simulink model "SVPWM"  (R2023b)
settings: Solver=FixedStepAuto  StartTime=0.0  StopTime=10.0  FixedStep=1e-4  RelTol=1e-3
values from neighbouring files (symbols this model uses):
  flux = 0.016884    [SVPWM.sldd]
  Period = 8000.0    [SVPWM.sldd]
  Pn = 4.0    [SVPWM.sldd]
  Udc = 24.0    [SVPWM.sldd]
libraries: mcbplantlib x1, autolibpmsmexterior x1
settings Model: DataDictionary=SVPWM.sldd  Creator=Administrator  LastModifiedBy=SkyLin
settings OptimizationCC: DefaultParameterBehavior=Inlined  UseDivisionForNetSlopeComputation=on  GainParamInheritBuiltInType=on  UseFloatMulNetSlope=on  InlineInvariantSignals=on  PassReuseOutputArgsAs=Individual arguments  ZeroExternalMemoryAtStartup=off  ZeroInternalMemoryAtStartup=off  NoFixptDivByZeroProtection=on  EfficientFloat2IntCast=on  LifeSpan=1  OptimizeBlockOrder=speed  DifferentSizesBufferReuse=on  EfficientTunableParamExpr=on
settings DebuggingCC: ParameterTunabilityLossMsg=error  UnconnectedInputMsg=warning  UnconnectedOutputMsg=warning  UnconnectedLineMsg=warning
settings HardwareCC: ProdBitPerPointer=32  ProdBitPerSizeT=32  ProdBitPerPtrDiffT=32  ProdLargestAtomicInteger=Long  ProdLargestAtomicFloat=Double  ProdWordSize=32  ProdLongLongMode=on  ProdHWDeviceType=ARM Compatible->ARM Cortex-M
settings ModelReferenceCC: EnableRefExpFcnMdlSchedulingChecks=on
settings SFSimCC: MATLABDynamicMemAlloc=off
settings RTWCC: Description=Embedded Coder  SystemTargetFile=ert.tlc  GenCodeOnly=on  TemplateMakefile=ert_default_tmf  GenerateReport=on  LaunchReport=on  GenerateCodeReplacementReport=on  DLArmComputeVersion=19.05
settings CodeAppCC: ForceParamTrailComments=on  IgnoreCustomStorageClasses=off  OperatorAnnotations=on  SimulinkDataObjDesc=on  SFDataObjDesc=on  CustomSymbolStrGlobalVar=rt$N$M  CustomSymbolStrType=$N$M  CustomSymbolStrFcn=$N$M$F  CustomSymbolStrMacro=$N$M  InsertBlockDesc=on
settings ERTTargetCC: TargetLangStandard=C99 (ISO)  CodeReplacementLibrary=ARM Cortex-M  GenerateSampleERTMain=on  IncludeMdlTerminateFcn=off  CombineSignalStateStructs=on  SuppressErrorStatus=on  SupportAbsoluteTime=off  SupportNonFinite=off  SupportComplex=off  InlinedParameterPlacement=NonHierarchical  ERTCustomFileTemplate=example_file_process.tlc  ERTFilePackagingFormat=CompactWithDataFile

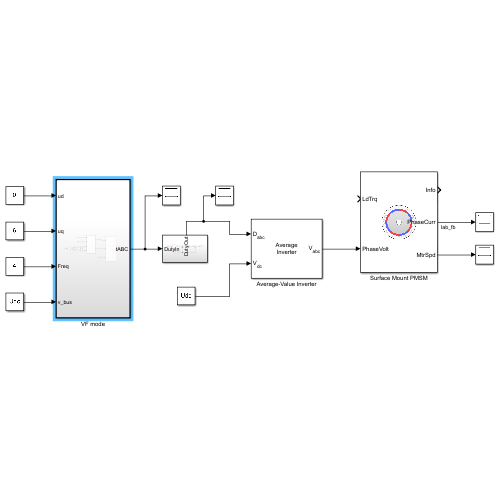
[thumbnail: Simulink's stored preview of the top-level diagram]
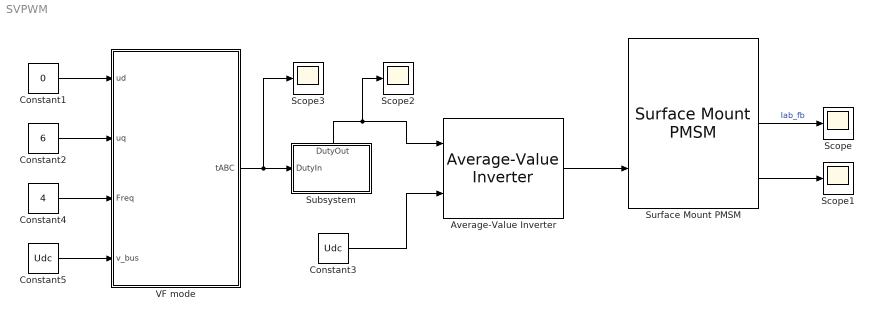
== system SVPWM ==
  Average-Value Inverter : mcbplantlib/Average-Value Inverter
  Constant1 : Constant  Value=0  OutDataTypeStr=single
  Constant2 : Constant  Value=6  OutDataTypeStr=single
  Constant3 : Constant  Value=Udc
  Constant4 : Constant  Value=4  OutDataTypeStr=single
  Constant5 : Constant  Value=Udc  OutDataTypeStr=single
  Scope{,1..3} (4 alike) : Scope
  Subsystem : Subsystem
      settings: PortSchema="{\"entries\":[{\"content\":{\"sides\":[{\"content\":{\"connectorIds\":[\"In1\"]},\"type\":\"ConnectorPlacement.EquallySpacedRectSide\",\"uuid\":\"8ccc51de-fa2a-4900-80a3-4cdf9aa76f01\"},{\"content\":{\"connectorIds\":[],\"side\":\"RIGHT\"},\"type\":\"ConnectorPlacement.EquallySpacedRectSide\",\"uuid\":\"32c06e0d-3f1d-4948-af96-e310e54308a0\"},{\"content\":{\"connectorIds\":[\"Out1\"],\"side\":\"TOP\"},\"type\":\"ConnectorPlacement.EquallySpacedRectSide\",\"uuid\":\"a9066067-2c54-42a8-b4d7-fb86ac71b860\"}]},\"type\":\"ConnectorPlacement.EquallySpacedConnector\",\"uuid\":\"e4576975-acad-4e16-822f-2c2e7f23d7a7\"}],\"packageUris\":[\"http://schema.mathworks.com/mf0/Connector/R2020b\"],\"version\":\"1.0\"}"
  Surface Mount PMSM : autolibpmsmexterior/Surface Mount PMSM  port_config=Torque  sim_type=Discrete  Ts=1e-4  P=Pn  Rs=Rs  Ldq_=L  KConstText=Permanent flux linkage constant (lambda_pm):  lambda_pm=flux  Ke=0.0059268  Kt=0.061  mechanical=[75e-6, 8e-5, 0]  idq0=[0 0]  theta_init=4/5  omega_init=0  KConst=flux  lambda_pm_calc=flux  RefBlkName='autolibpmsmexterior/Surface Mount PMSM'  aMode=5  Ldq="[0.0017      0.0017]"
  VF mode : Subsystem  TreatAsAtomicUnit=on
      settings: RTWSystemCode=Nonreusable function
  wires:
  VF mode/1(tABC) -> Scope3/1, Subsystem/1(DutyIn)
  Constant3/1 -> Average-Value Inverter/2
  Subsystem/1(DutyOut) -> Scope2/1, Average-Value Inverter/1
  Average-Value Inverter/1 -> Surface Mount PMSM/2
  Surface Mount PMSM/2 -> Scope/1  "Iab_fb"
  Surface Mount PMSM/3 -> Scope1/1
  Constant1/1 -> VF mode/1(ud)
  Constant2/1 -> VF mode/2(uq)
  Constant4/1 -> VF mode/3(Freq)
  Constant5/1 -> VF mode/4(v_bus)

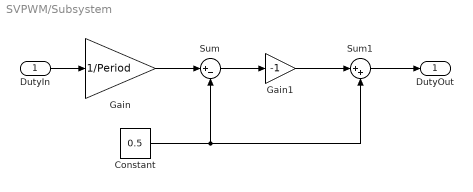
== system SVPWM/Subsystem ==
  DutyIn : Inport
  Constant : Constant  Value=0.5  SampleTime=-1
  Gain : Gain  Gain=1/Period  ParamDataTypeStr=single
  Gain1 : Gain  Gain=-1
  Sum : Sum  Inputs=|+-
  Sum1 : Sum  Inputs=|++
  DutyOut : Outport
  wires:
  Sum/1 -> Gain1/1
  Constant/1 -> Sum1/2, Sum/2
  DutyIn/1 -> Gain/1
  Gain1/1 -> Sum1/1
  Sum1/1 -> DutyOut/1
  Gain/1 -> Sum/1

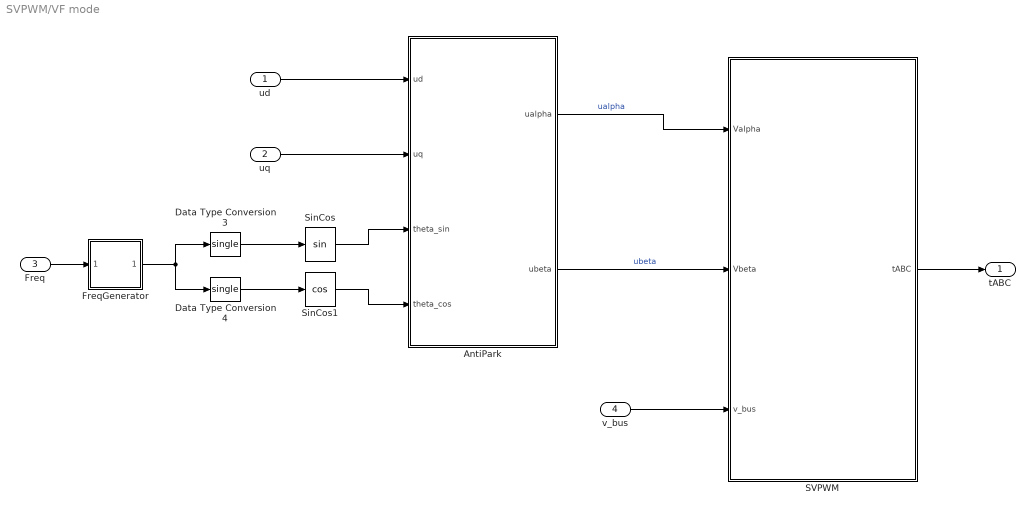
== system SVPWM/VF mode ==
  ud : Inport
  uq : Inport  Port=2
  Freq : Inport  Port=3
  v_bus : Inport  Port=4
  AntiPark : Subsystem
  Data Type Conversion3 : DataTypeConversion  OutDataTypeStr=single  SaturateOnIntegerOverflow=off  RndMeth=Floor
  Data Type Conversion4 : DataTypeConversion  OutDataTypeStr=single  SaturateOnIntegerOverflow=off  RndMeth=Floor
  FreqGenerator : Subsystem
  SVPWM : Subsystem  TreatAsAtomicUnit=on
  SinCos : Trigonometry
  SinCos1 : Trigonometry  Operator=cos
  tABC : Outport
  wires:
  FreqGenerator/1(Theta) -> Data Type Conversion4/1, Data Type Conversion3/1
  SinCos1/1 -> AntiPark/4(theta_cos)
  Data Type Conversion4/1 -> SinCos1/1
  SinCos/1 -> AntiPark/3(theta_sin)
  Freq/1 -> FreqGenerator/1(Freq)
  Data Type Conversion3/1 -> SinCos/1
  AntiPark/1(ualpha) -> SVPWM/1(Valpha)  "ualpha"
  AntiPark/2(ubeta) -> SVPWM/2(Vbeta)  "ubeta"
  ud/1 -> AntiPark/1(ud)
  uq/1 -> AntiPark/2(uq)
  v_bus/1 -> SVPWM/3(v_bus)
  SVPWM/1(tABC) -> tABC/1

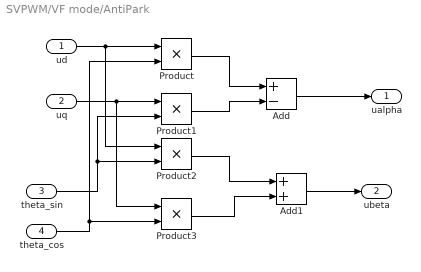
== system SVPWM/VF mode/AntiPark ==
  ud : Inport
  uq : Inport  Port=2
  theta_sin : Inport  Port=3
  theta_cos : Inport  Port=4
  Add : Sum  Inputs=+-
  Add1 : Sum
  Product{,1..3} (4 alike) : Product
  ualpha : Outport  OutDataTypeStr=single
  ubeta : Outport  Port=2  OutDataTypeStr=single
  wires:
  Add1/1 -> ubeta/1
  Product1/1 -> Add/2
  uq/1 -> Product3/1, Product1/1
  theta_cos/1 -> Product/2, Product3/2
  theta_sin/1 -> Product2/2, Product1/2
  ud/1 -> Product2/1, Product/1
  Product3/1 -> Add1/2
  Add/1 -> ualpha/1
  Product/1 -> Add/1
  Product2/1 -> Add1/1

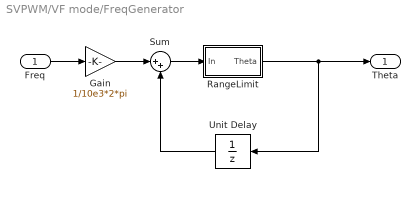
== system SVPWM/VF mode/FreqGenerator ==
  Freq : Inport
  Gain : Gain  Gain=1/10e3*2*pi  OutDataTypeStr=single
  RangeLimit : Subsystem
  Sum : Sum  Inputs=|++  OutDataTypeStr=Inherit: Same as first input
  Unit Delay : UnitDelay  SampleTime=-1  HasFrameUpgradeWarning=on
  Theta : Outport
  wires:
  Freq/1 -> Gain/1
  RangeLimit/1(Theta) -> Theta/1, Unit Delay/1
  Gain/1 -> Sum/1
  Sum/1 -> RangeLimit/1(In)
  Unit Delay/1 -> Sum/2

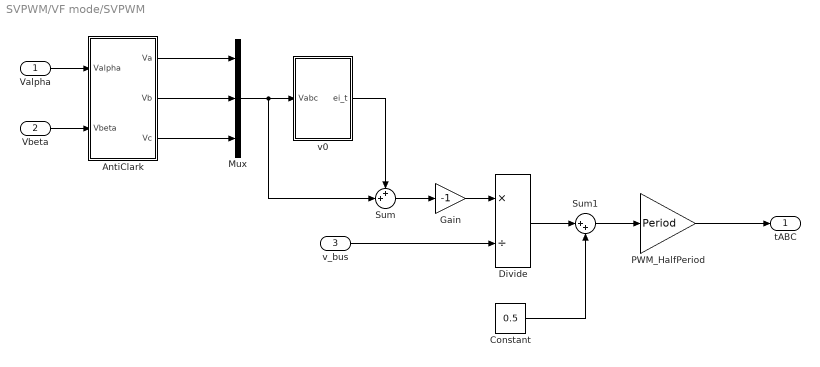
== system SVPWM/VF mode/SVPWM ==
  Valpha : Inport  OutDataTypeStr=single
  Vbeta : Inport  Port=2  OutDataTypeStr=single
  v_bus : Inport  Port=3  OutDataTypeStr=single
  AntiClark : Subsystem
  Constant : Constant  Value=0.5  OutDataTypeStr=single
  Divide : Product  Inputs=*/  OutDataTypeStr=single
  Gain : Gain  Gain=-1  OutDataTypeStr=single
  Mux : Mux  Inputs=3
  PWM_HalfPeriod : Gain  Gain=Period  OutDataTypeStr=single
  Sum : Sum  Inputs=++|  OutDataTypeStr=single
  Sum1 : Sum  Inputs=|++  OutDataTypeStr=single
  v0 : Subsystem
  tABC : Outport  OutDataTypeStr=single
  wires:
  Valpha/1 -> AntiClark/1(Valpha)
  Vbeta/1 -> AntiClark/2(Vbeta)
  v0/1(ei_t) -> Sum/1
  AntiClark/1(Va) -> Mux/1
  AntiClark/2(Vb) -> Mux/2
  AntiClark/3(Vc) -> Mux/3
  Sum/1 -> Gain/1
  Mux/1 -> Sum/2, v0/1(Vabc)
  Divide/1 -> Sum1/1
  Constant/1 -> Sum1/2
  Sum1/1 -> PWM_HalfPeriod/1
  PWM_HalfPeriod/1 -> tABC/1
  v_bus/1 -> Divide/2
  Gain/1 -> Divide/1

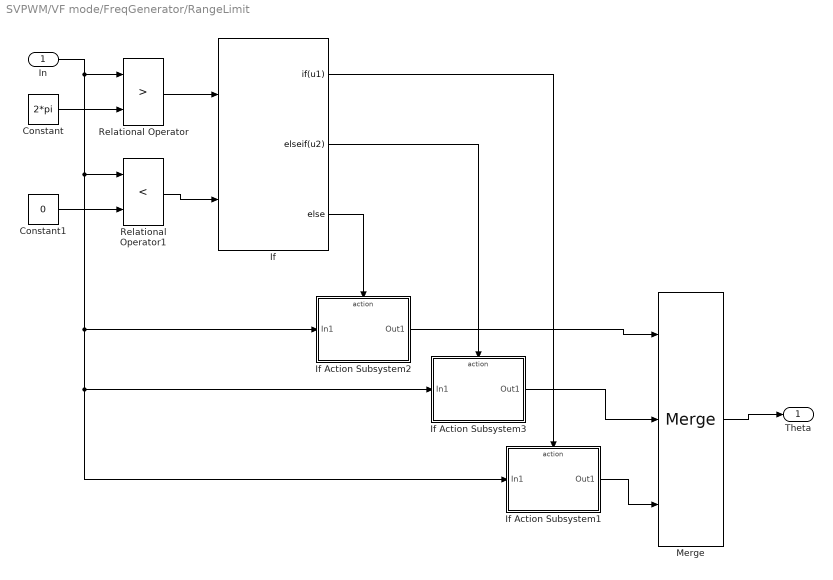
== system SVPWM/VF mode/FreqGenerator/RangeLimit ==
  In : Inport
  Constant : Constant  Value=2*pi  OutDataTypeStr=single  SampleTime=-1
  Constant1 : Constant  Value=0  OutDataTypeStr=single  SampleTime=-1
  If : If  NumInputs=2  IfExpression=u1  ElseIfExpressions=u2
  If Action Subsystem1 : Subsystem  TreatAsAtomicUnit=on
  If Action Subsystem2 : Subsystem  TreatAsAtomicUnit=on
  If Action Subsystem3 : Subsystem  TreatAsAtomicUnit=on
  Merge : Merge  Inputs=3
  Relational Operator : RelationalOperator  Operator=>  OutDataTypeStr=boolean  RndMeth=Simplest  InputSameDT=off
  Relational Operator1 : RelationalOperator  Operator=<  OutDataTypeStr=boolean  RndMeth=Simplest  InputSameDT=off
  Theta : Outport
  wires:
  Relational Operator/1 -> If/1
  Constant/1 -> Relational Operator/2
  In/1 -> Relational Operator1/1, If Action Subsystem2/1(In1), If Action Subsystem3/1(In1), If Action Subsystem1/1(In1), Relational Operator/1
  Merge/1 -> Theta/1
  If/3 -> If Action Subsystem2/Action
  If/1 -> If Action Subsystem1/Action
  If Action Subsystem2/1(Out1) -> Merge/1
  Constant1/1 -> Relational Operator1/2
  Relational Operator1/1 -> If/2
  If/2 -> If Action Subsystem3/Action
  If Action Subsystem1/1(Out1) -> Merge/3
  If Action Subsystem3/1(Out1) -> Merge/2

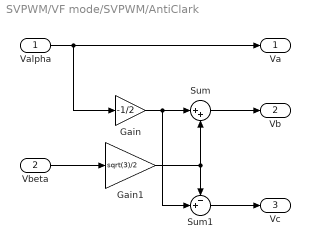
== system SVPWM/VF mode/SVPWM/AntiClark ==
  Valpha : Inport  OutDataTypeStr=single
  Vbeta : Inport  Port=2  OutDataTypeStr=single
  Gain : Gain  Gain=-1/2  OutDataTypeStr=single
  Gain1 : Gain  Gain=sqrt(3)/2  OutDataTypeStr=single
  Sum : Sum  Inputs=|++  OutDataTypeStr=single
  Sum1 : Sum  Inputs=-+|  OutDataTypeStr=single
  Va : Outport  OutDataTypeStr=single
  Vb : Outport  Port=2  OutDataTypeStr=single
  Vc : Outport  Port=3  OutDataTypeStr=single
  wires:
  Valpha/1 -> Gain/1, Va/1
  Vbeta/1 -> Gain1/1
  Gain/1 -> Sum1/2, Sum/1
  Sum/1 -> Vb/1
  Gain1/1 -> Sum/2, Sum1/1
  Sum1/1 -> Vc/1

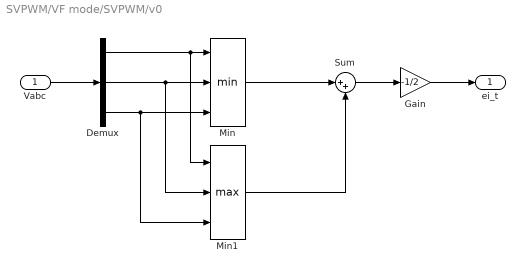
== system SVPWM/VF mode/SVPWM/v0 ==
  Vabc : Inport  OutDataTypeStr=single
  Demux : Demux  Outputs=3
  Gain : Gain  Gain=-1/2  OutDataTypeStr=single
  Min : MinMax  Inputs=3  OutDataTypeStr=single
  Min1 : MinMax  Function=max  Inputs=3  OutDataTypeStr=single
  Sum : Sum  Inputs=|++  OutDataTypeStr=single
  ei_t : Outport  OutDataTypeStr=single
  wires:
  Min/1 -> Sum/1
  Sum/1 -> Gain/1
  Min1/1 -> Sum/2
  Gain/1 -> ei_t/1
  Vabc/1 -> Demux/1
  Demux/1 -> Min1/1, Min/1
  Demux/2 -> Min/2, Min1/2
  Demux/3 -> Min1/3, Min/3

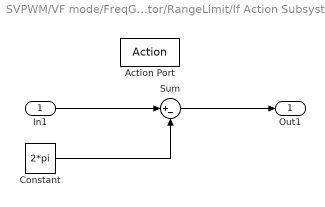
== system SVPWM/VF mode/FreqGenerator/RangeLimit/If Action Subsystem1 ==
  In1 : Inport
  Action Port : ActionPort  ActionPortLabel=if(u1)
  Constant : Constant  Value=2*pi  OutDataTypeStr=single  SampleTime=-1
  Sum : Sum  Inputs=|+-
  Out1 : Outport
  wires:
  In1/1 -> Sum/1
  Constant/1 -> Sum/2
  Sum/1 -> Out1/1

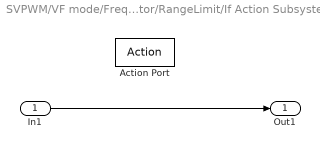
== system SVPWM/VF mode/FreqGenerator/RangeLimit/If Action Subsystem2 ==
  In1 : Inport
  Action Port : ActionPort  ActionPortLabel=else
  Out1 : Outport
  wires:
  In1/1 -> Out1/1

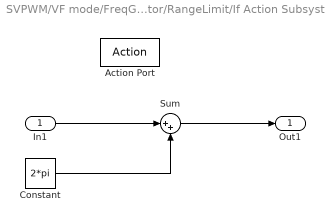
== system SVPWM/VF mode/FreqGenerator/RangeLimit/If Action Subsystem3 ==
  In1 : Inport
  Action Port : ActionPort  ActionPortLabel=elseif(u2)
  Constant : Constant  Value=2*pi  OutDataTypeStr=single  SampleTime=-1
  Sum : Sum  Inputs=|++
  Out1 : Outport
  wires:
  Constant/1 -> Sum/2
  In1/1 -> Sum/1
  Sum/1 -> Out1/1
